simulink model "videoViewer"  (R2013b)
settings: Solver=FixedStepDiscrete  StartTime=0.0  StopTime=inf  RelTol=1e-3
undefined symbols (not defined in the file or in its folder): gray
libraries: xpcvideoutillib x2, xpclib x1, visionsinks x1
settings Model: xpc_rtwmakecfg_data=_jpeg_  BufferReuse=off  Creator=gweast  LastModifiedBy=Doctor V
settings DataIOCC: LimitDataPoints=off  SignalLoggingSaveFormat=ModelDataLogs
settings OptimizationCC: BlockReduction=off  OptimizeBlockIOStorage=off  BufferReuse=off  ExpressionFolding=off  ExpressionDepthLimit=2147483647  LocalBlockOutputs=off  SimCompilerOptimization=On
settings DebuggingCC: InheritedTsInSrcMsg=none  FcnCallInpInsideContextMsg=UseLocalSettings  StateNameClashWarn=warning
settings HardwareCC: ProdIntDivRoundTo=Zero  ProdEndianess=LittleEndian  ProdHWDeviceType=Generic->32-bit x86 compatible
settings RTWCC: SystemTargetFile=xpctarget.tlc  TemplateMakefile=xpc_default_tmf  Description=xPC Target  ProcessScript=xpctarget_make_rtw_hook  RTWCompilerOptimization=On
settings xpcTargetCC: TargetFcnLib=ansi_tfl_table_tmw.mat  CodeReplacementLibrary=XPC_BLAS  ParMdlRefBuildCompliant=on  ConcurrentExecutionCompliant=on  CombineSignalStateStructs=off  MATLABClassNameForMDSCustomization=xpcAperiodicCustomization  GRTInterface=on  GenerateAllocFcn=off  RL32LogBufSizeModifier=1000000000000  xPCTaskExecutionProfile=off  xPCRL32EventNumber=50000000000  xPCLoadParamSetFile=off  xPCConcurrentTasks=off  xPCEnableSFAnimation=off

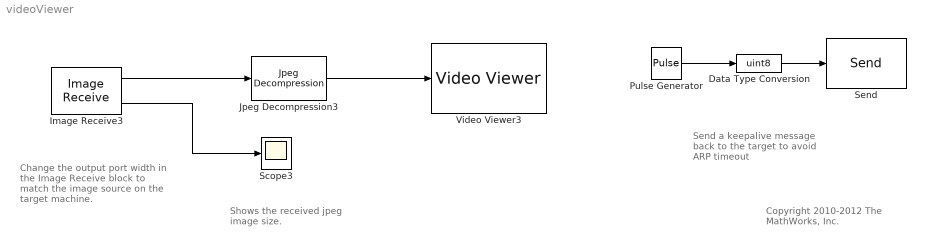
== system videoViewer ==
  note: Send a keepalive message back
      | to the target to avoid ARP timeout
  note: Copyright 2010-2012 The MathWorks, Inc.
  note: Shows the received
      | jpeg image size.
  note: Change the output port width
      | in the Image Receive block to
      | match the image source on the
      | target machine.
  Data Type Conversion : DataTypeConversion  OutDataTypeStr=uint8
  Image Receive3 : xpcvideoutillib/Image Receive  ipAddress=0.0.0.0  ipPort=25000  width=2040*1088  vblLen=on  maxpacket=40*1024  sampletime=1/30
  Jpeg Decompression3 : xpcvideoutillib/Jpeg Decompression  width=2040  height=1088  cspace=Grayscale  isig=One multidimensional signal  trigger=off
  Pulse Generator : DiscretePulseGenerator  Period=10  PulseWidth=5  SampleTime=-1
  Scope3 : Scope
      settings: TimeRange=4  YMin=0  YMax=80000
  Send : xpclib/UDP/Send  ipAddress=10.10.10.12  ipPort=-1  localPort=-1  vblLen=off  sampletime=-1
  Video Viewer3 : visionsinks/Video Viewer  inputType=Obsolete7b  imagePorts=One multidimensional signal  useColorMap=off  colormapValue=gray(256)  specRange=off  minInputVal=0  maxInputVal=255  FigPos=[-2263 678 1046 540]  AxisZoom=on  trueSizedOnce=off  OpenAtMdlStart=on  DefaultConfigurationName=vipscopes.VideoViewerScopeCfg
  wires:
  Pulse Generator/1 -> Data Type Conversion/1
  Data Type Conversion/1 -> Send/1
  Image Receive3/2 -> Scope3/1
  Image Receive3/1 -> Jpeg Decompression3/1
  Jpeg Decompression3/1 -> Video Viewer3/1
